simulink model "q5_hw7"  (R2021b)
settings: Solver=VariableStepAuto  StartTime=0.0  StopTime=40  RelTol=1e-3
values from neighbouring files (symbols this model uses):
  K = (3*s^2+3.3*s+0.3)/(s^2+0.3*s)    [q1.m]    (also in q2.m = Xs/Ys; q4.m = Xs/Ys; q5.m = K/(s*(s^2+4)))
libraries: simulink x1
settings Model: Creator=Reyhaneh  LastModifiedBy=Reyhaneh

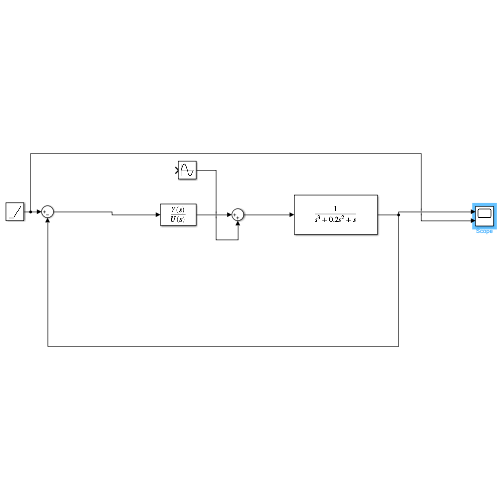
[thumbnail: Simulink's stored preview of the top-level diagram]
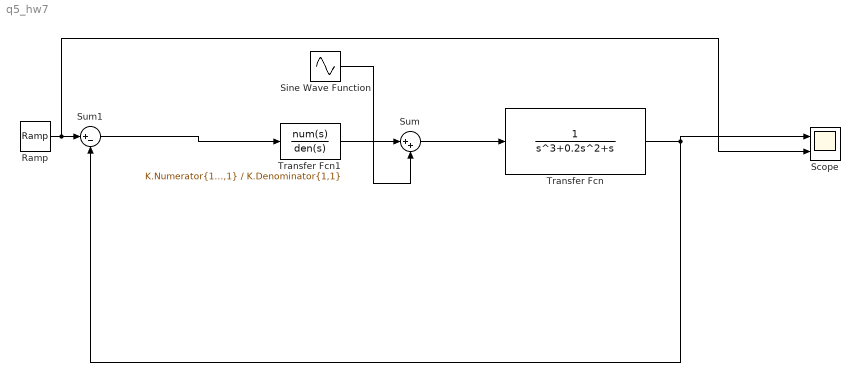
== system q5_hw7 ==
  Ramp : simulink/Sources/Ramp  slope=1  start=0  InitialOutput=0
  Scope : Scope  NumInputPorts=2
  Sine Wave Function : Sin  TimeSource=Use external signal  Frequency=2  SampleTime=0
  Sum : Sum  Inputs=|++
  Sum1 : Sum  Inputs=|+-
  Transfer Fcn : TransferFcn  Denominator=[1 0.2 1 0]
  Transfer Fcn1 : TransferFcn  Numerator=K.Numerator{1,1}  Denominator=K.Denominator{1,1}
  wires:
  Transfer Fcn/1 -> Sum1/2, Scope/1
  Ramp/1 -> Scope/2, Sum1/1
  Sum1/1 -> Transfer Fcn1/1
  Sine Wave Function/1 -> Sum/2
  Transfer Fcn1/1 -> Sum/1
  Sum/1 -> Transfer Fcn/1
